simulink model "tesys_original"  (R2020b)
settings: Solver=VariableStepAuto  StartTime=0.0  StopTime=100  RelTol=1e-3
values from neighbouring files (symbols this model uses):
  chisqResidualExp = [0.0306450479532 0.0531264498325 0.923642363871 -0.0297874458631 -0.514662448138 -0.00656924053761 -0.0063391426586 0.00645293061692 -0.0736933231173 -0.060106090774 -0.0130451403889 -0.410405834788 ... (256 elements, 16x16)]    [basevars_performanceTests.mat]
  NoiseVariance = [0.018084969162 0.0123441994291 0.623950185025 -0.0183166694842 -0.436214576367 -0.00523694618209 -0.007053197837 0.0054321930422 -0.0564553252382 -0.0606906681254 -0.0118460528722 -0.365322092979 ... (256 elements, 16x16)]    [basevars_performanceTests.mat]
  threshold = 25.9894230826    [basevars_performanceTests.mat]
  u0 = [63.053 53.98 24.644 61.302 22.21 40.064 38.1 46.534 47.446 41.106 18.114 50]    [basevars_performanceTests.mat]
  y0 = [0.250521392428 3664.03885069 4509.26819729 9.3477426267 2704.99998425 74.9999967369 120.399999605 0.337117068415 80.1094039946 50.0000005823 25.1601724781 49.9999996443 ... (16 elements, 16x1)]    [basevars_performanceTests.mat]
undefined symbols (not defined in the file or in its folder): Discrete, sigbuilder_block, ssid_est, ssid_estred, Time
libraries: TElib x17, simulink x1, truetime x1, ctrlSharedLib x1
settings Model: Creator=mazen  LastModifiedBy=mazen
settings DataIOCC: InitialState=xInitialTecode  SaveOperatingPoint=on  SaveFormat=Structure  SaveOutput=off  SaveState=on  SignalLogging=off  DSMLogging=off

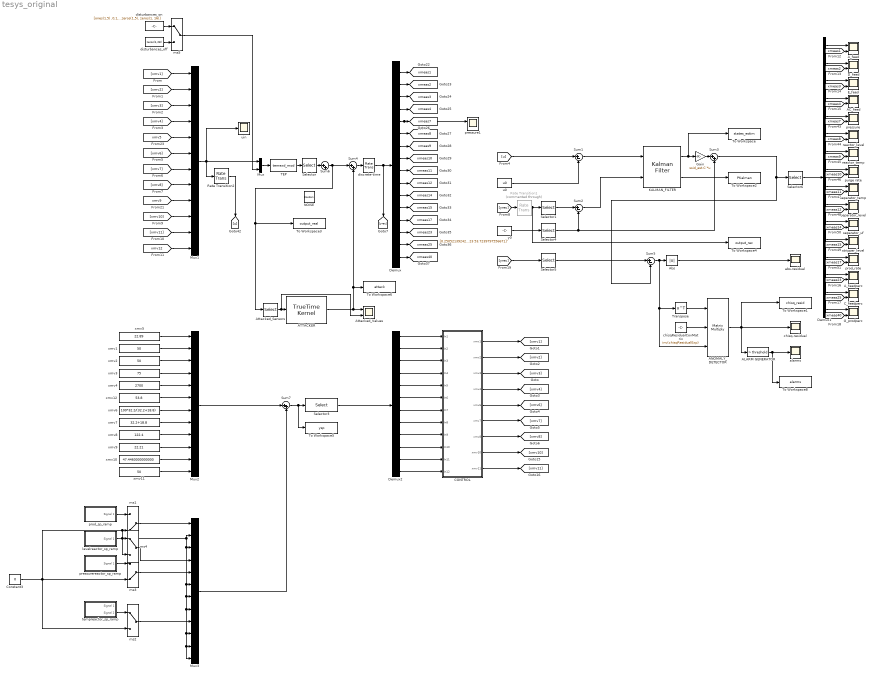
== system tesys_original ==
  AC_feed : Scope  NumInputPorts=2
  ALARM GENERATOR : simulink/Logic and Bit Operations/Compare To Constant  relop=>  const=threshold  OutDataTypeStr=boolean
  ANOMALY_DETECTOR : Product  Inputs=3  Multiplication=Matrix(*)
  ATTACKER : truetime/TrueTime Kernel  sfun=attacker_init  args="struct('FalseAlarmRate',0.1,'Start',20,'AttackedSensors',[5   6   7   9  10  12],'AttackCoef',0.0049316)"  ninputsoutputs=[6 16]  ntriggers=0  trigtype=falling  nwnodenbr=[]  clockoffsetdrift=[0 0]  schedoutput=off  battery=off  poweroutput=off
  A_feed : Scope  NumInputPorts=2
  A_feedperc : Scope  NumInputPorts=2
  Abs : Abs  ZeroCross=off
  Attacked_Sensors : Selector  InputPortWidth=16  IndexOptions=Index vector (dialog)  Indices="[5   6   7   9  10  12]"  OutputSizes=1
  Attacked_Values : Scope  NumInputPorts=2
  CONTROL : Subsystem
  C_feedperc : Scope  NumInputPorts=2
  Constant3 : Constant  Value=0
  D_feed : Scope  NumInputPorts=2
  Demux : Demux  Outputs=16
      settings: DisplayOption=none
  Demux1 : Demux  Outputs=16
      settings: DisplayOption=none
  Demux2 : Demux  Outputs=12
  E_feed : Scope  NumInputPorts=2
  G_prodperc : Scope  NumInputPorts=2
  Gain : Gain  Gain=ssid_est.C  Multiplication=Matrix(K*u)
  KALMAN_FILTER : ctrlSharedLib/Kalman Filter  TimeDomain=Discrete-Time  UseCurrentEstimator=off  ModelSource=LTI State-Space Variable  ModelSourceVariable=ssid_est  A=0.95  B=1  C=1  D=0  NumberOfStates=1  NumberOfInputs=1  NumberOfOutputs=1  InitialEstimateSource=Dialog  X0=0  P0=10  UseK=off  UseGH=off  NumberOfProcessNoiseInputs=1  G=eye(size(ssid_estred.A,1))  TimeInvariantG=on  H=zeros(16,50)  TimeInvariantH=on  Q=diag(ones(size(ssid_est.A,1),1))  TimeInvariantQ=on  R=NoiseVariance  TimeInvariantR=on  N=0  TimeInvariantN=on  AddInputPort=on  AddEnablePort=off  OutputEstimatedY=off  OutputP=on  Ts=-1
      link override MemoryX: InitialCondition="[0.011146   -0.044581   -0.057523    0.064041    0.011425    -0.12859    0.010301   -0.022916    -0.07193   -0.023009   -0.055426    0.037347    0.028076    0.037152    -0.03861     0.02741   -0.018561    0.069301    0.039131   -0.021743   0.0059364    0.075828    0.041172    0.018942   -0.016117     0.12945    -0.05531   -0.047396    0.003457  0.00092852   0.0034323  -0.0053009  6.7113e-05   0.0047184   0.0075023  -0.0024375    0.015481   -0.008098   0.0051102    0.004456    0.010581  -0.0041833     0.02045   -0.015462  -0.0080483   -0.010569  -0.0081562    0.041485    -0.02002    0.026945]"
  Mux : Mux  Inputs=2
  Mux1 : Mux  Inputs=12
  Mux2 : Mux  Inputs=12
  Mux3 : Mux  Inputs=12
  NOISE : RandomNumber  Variance=0.001*y0  SampleTime=5e-4
  Rate Transition1 : RateTransition  Commented=through  InitialCondition=y0  OutPortSampleTime=5e-4
  Rate Transition2 : RateTransition  OutPortSampleTime=5e-4
  Selector : Selector  InputPortWidth=41  IndexOptions=Index vector (dialog)  Indices=[1:4, 7:12, 14, 15, 17, 23, 25, 40]  OutputSizes=1
  Selector1 : Selector  InputPortWidth=16  IndexOptions=Index vector (dialog)  Indices=y0_selected  OutputSizes=1
  Selector3 : Selector  InputPortWidth=12  IndexOptions=Index vector (dialog)  Indices=[1,6,7,8,5,3,2,9,4,10,11,12]  OutputSizes=1
  Selector4 : Selector  InputPortWidth=16  IndexOptions=Index vector (dialog)  Indices=y0_selected  OutputSizes=1
  Selector5 : Selector  InputPortWidth=16  IndexOptions=Index vector (dialog)  Indices=y0_selected  OutputSizes=1
  Selector6 : Selector  InputPortWidth=16  IndexOptions=Index vector (dialog)  Indices=y0_selectedinv  OutputSizes=1
  Sum1 : Sum  Inputs=|+-
  Sum2 : Sum  Inputs=|+-
  Sum{3..4,6..7} (4 alike) : Sum  Inputs=|++
  Sum5 : Sum  Inputs=|+-
  TEP : S-Function  FunctionName=temexd_mod  Parameters=[],[], 0  SFunctionDeploymentMode=off  EnableBusSupport=off
  To Workspace : ToWorkspace  VariableName=states_estim  SampleTime=0.01
  To Workspace1 : ToWorkspace  VariableName=chisq_resid  SampleTime=0.01
  To Workspace2 : ToWorkspace  VariableName=PKalman  SampleTime=0.01
  To Workspace3 : ToWorkspace  VariableName=output_real  SampleTime=0.01
  To Workspace4 : ToWorkspace  VariableName=output_rec  SampleTime=0.01
  To Workspace5 : ToWorkspace  VariableName=ysp  SampleTime=0.01
  To Workspace6 : ToWorkspace  VariableName=attack  SampleTime=5e-4
  To Workspace8 : ToWorkspace  VariableName=alarms  SampleTime=5e-4
  Transpose : Math  Operator=transpose  SaturateOnIntegerOverflow=on
  abs-residual : Scope
  alarms : Scope
  chisq-residual : Scope
  chisqResidualCovMatrix : Constant  Value=inv(chisqResidualExp)
  discrete-time : RateTransition  OutPortSampleTime=5e-4
  disturbances_off : Constant  Value=zeros(1,28)
  disturbances_on : Constant  Value=[ones(1,5) ,0,1,zeros(1,5), zeros(1, 16)]
  levelreactor_sp_ramp : Subsystem  Tag=STV Subsys  LoadFcn=sigbuilder_block('load');  StartFcn=sigbuilder_block('start');  StopFcn=sigbuilder_block('stop');  ClipboardFcn=sigbuilder_block('clipboard');  mask(Sigbuilder block){tuvar=[0:10]}
      mask help: Simulink:masks:SigbuilderBlock_MD
      mask init:
      | if ~strcmp(get_param(bdroot(gcbh),'SimulationStatus'),'stopped') tuvar = sigbuilder_block('maskInit'); end
      settings: CopyFcn=sigbuilder_block('copy');  DeleteFcn=sigbuilder_block('delete');  ModelCloseFcn=sigbuilder_block('modelClose');  PreSaveFcn=sigbuilder_block('preSave');  PauseFcn=sigbuilder_block('pause');  ContinueFcn=sigbuilder_block('continue');  NameChangeFcn=sigbuilder_block('namechange');  OpenFcn=sigbuilder_block('open',[437.6 199.2 550.4 400 ]);  CloseFcn=sigbuilder_block('close');
      mask Display: plot(0, 0, 100, 100,[2, 2, 32, 32, 2], [68, 8, 8, 68, 68],[32, 2], [38, 38], [32, 19, 2],[53, 60, 44], [32, 17, 17, 2],[16, 16, 31, 31]);txt = getActiveGroup(gcbh);text(2, 100, txt,'verticalAlignment', 'top');
  ms1 : ManualSwitch  CurrentSetting=0
  ms2 : ManualSwitch
  ms3 : ManualSwitch  CurrentSetting=0
  ms4 : ManualSwitch
  ms5 : ManualSwitch
  pressure : Scope  NumInputPorts=2
  pressure1 : Scope  NumInputPorts=2
  pressurereactor_sp_ramp : Subsystem  Tag=STV Subsys  LoadFcn=sigbuilder_block('load');  StartFcn=sigbuilder_block('start');  StopFcn=sigbuilder_block('stop');  ClipboardFcn=sigbuilder_block('clipboard');  mask(Sigbuilder block){tuvar=[0:10]}
      mask help: Simulink:masks:SigbuilderBlock_MD
      mask init:
      | if ~strcmp(get_param(bdroot(gcbh),'SimulationStatus'),'stopped') tuvar = sigbuilder_block('maskInit'); end
      settings: CopyFcn=sigbuilder_block('copy');  DeleteFcn=sigbuilder_block('delete');  ModelCloseFcn=sigbuilder_block('modelClose');  PreSaveFcn=sigbuilder_block('preSave');  PauseFcn=sigbuilder_block('pause');  ContinueFcn=sigbuilder_block('continue');  NameChangeFcn=sigbuilder_block('namechange');  OpenFcn=sigbuilder_block('open',[437.6 199.2 550.4 400 ]);  CloseFcn=sigbuilder_block('close');
      mask Display: plot(0, 0, 100, 100,[2, 2, 32, 32, 2], [68, 8, 8, 68, 68],[32, 2], [38, 38], [32, 19, 2],[53, 60, 44], [32, 17, 17, 2],[16, 16, 31, 31]);txt = getActiveGroup(gcbh);text(2, 100, txt,'verticalAlignment', 'top');
  prod_rate : Scope  NumInputPorts=2
  prod_sp_ramp : Subsystem  Tag=STV Subsys  LoadFcn=sigbuilder_block('load');  StartFcn=sigbuilder_block('start');  StopFcn=sigbuilder_block('stop');  ClipboardFcn=sigbuilder_block('clipboard');  mask(Sigbuilder block){tuvar=[0:10]}
      mask help: Simulink:masks:SigbuilderBlock_MD
      mask init:
      | if ~strcmp(get_param(bdroot(gcbh),'SimulationStatus'),'stopped') tuvar = sigbuilder_block('maskInit'); end
      settings: CopyFcn=sigbuilder_block('copy');  DeleteFcn=sigbuilder_block('delete');  ModelCloseFcn=sigbuilder_block('modelClose');  PreSaveFcn=sigbuilder_block('preSave');  PauseFcn=sigbuilder_block('pause');  ContinueFcn=sigbuilder_block('continue');  NameChangeFcn=sigbuilder_block('namechange');  OpenFcn=sigbuilder_block('open',[437.6 199.2 550.4 400 ]);  CloseFcn=sigbuilder_block('close');
      mask Display: plot(0, 0, 100, 100,[2, 2, 32, 32, 2], [68, 8, 8, 68, 68],[32, 2], [38, 38], [32, 19, 2],[53, 60, 44], [32, 17, 17, 2],[16, 16, 31, 31]);txt = getActiveGroup(gcbh);text(2, 100, txt,'verticalAlignment', 'top');
  purge rate : Scope  NumInputPorts=2
  reactor_level : Scope  NumInputPorts=2
  reactor_temp : Scope  NumInputPorts=2
  separator_level : Scope  NumInputPorts=2
  separator_temp : Scope  NumInputPorts=2
  separator_uf : Scope  NumInputPorts=2
  stripper_level : Scope  NumInputPorts=2
  tempreactor_sp_ramp : Subsystem  Tag=STV Subsys  LoadFcn=sigbuilder_block('load');  StartFcn=sigbuilder_block('start');  StopFcn=sigbuilder_block('stop');  ClipboardFcn=sigbuilder_block('clipboard');  mask(Sigbuilder block){tuvar=[0:10]}
      mask help: Simulink:masks:SigbuilderBlock_MD
      mask init:
      | if ~strcmp(get_param(bdroot(gcbh),'SimulationStatus'),'stopped') tuvar = sigbuilder_block('maskInit'); end
      settings: CopyFcn=sigbuilder_block('copy');  DeleteFcn=sigbuilder_block('delete');  ModelCloseFcn=sigbuilder_block('modelClose');  PreSaveFcn=sigbuilder_block('preSave');  PauseFcn=sigbuilder_block('pause');  ContinueFcn=sigbuilder_block('continue');  NameChangeFcn=sigbuilder_block('namechange');  OpenFcn=sigbuilder_block('open',[437.6 199.2 550.4 400 ]);  CloseFcn=sigbuilder_block('close');
      mask Display: plot(0, 0, 100, 100,[2, 2, 32, 32, 2], [68, 8, 8, 68, 68],[32, 2], [38, 38], [32, 19, 2],[53, 60, 44], [32, 17, 17, 2],[16, 16, 31, 31]);txt = getActiveGroup(gcbh);text(2, 100, txt,'verticalAlignment', 'top');
  u0 : Constant  Value=u0  VectorParams1D=off
  "uin " : Scope
  xmv1 : Constant  Value=50
  xmv10 : Constant  Value=47.4460000000000
  xmv11 : Constant  Value=50
  xmv12 : Constant  Value=53.8
  xmv2 : Constant  Value=50
  xmv3 : Constant  Value=75
  xmv4 : Constant  Value=2700
  xmv5 : Constant  Value=22.89
  xmv6 : Constant  Value=100*32.2/(32.2+18.8)
  xmv7 : Constant  Value=32.2+18.8
  xmv8 : Constant  Value=122.4
  xmv9 : Constant  Value=22.21
  y0 : Constant  Value="[0.250521392427743\t3664.03885068600\t4509.26819729219\t9.34774262670434\t2704.99998424633\t74.9999967369169\t120.399999605037\t0.337117068414812\t80.1094039945582\t50.0000005822578\t25.1601724780539\t49.9999996443422\t22.9487308033689\t32.1876133826046\t26.3832900314723\t53.7239797556671]'"
  tag scope: xmeas10=global, xmeas11=global, xmeas12=global, xmeas14=global, xmeas15=global, xmeas17=global, xmeas1=global, xmeas23=global, xmeas25=global, xmeas2=global, xmeas3=global, xmeas40=global, xmeas4=global, xmeas7=global, xmeas8=global, xmeas9=global
  wires:
  [xmeas14] -> separator_uf/2
  [xmv11] -> Mux1/11
  [xmeas15] -> stripper_level/2
  [xmeas8] -> reactor_level/2
  [xmeas10] -> purge rate/2
  [xmeas11] -> separator_temp/2
  Demux/7 -> [xmeas9]
  Demux/5 -> pressure1/1, [xmeas7]
  Demux/9 -> [xmeas11]
  [xmeas12] -> separator_level/2
  [xmeas9] -> reactor_temp/2
  Sum6/1 -> Sum4/1, To Workspace3/1, Attacked_Sensors/1
  [xmv1] -> Mux1/1
  [xmv7] -> Mux1/7
  discrete-time/1 -> Demux/1, [yrec]
  [xmv10] -> Mux1/10
  [xmv8] -> Mux1/8
  [xmv6] -> Mux1/6
  Demux/6 -> [xmeas8]
  TEP/1 -> Selector/1
  [xmv5] -> Mux1/5
  [xmv3] -> Mux1/3
  [xmv4] -> Mux1/4
  Mux/1 -> TEP/1
  [xmeas7] -> pressure/2
  [xmeas17] -> prod_rate/2
  [xmv2] -> Mux1/2
  Demux/16 -> [xmeas40]
  Demux/15 -> [xmeas25]
  Demux/13 -> [xmeas17]
  Demux/11 -> [xmeas14]
  Demux/1 -> [xmeas1]
  Demux/3 -> [xmeas3]
  Demux/10 -> [xmeas12]
  u0/1 -> Sum1/2
  Demux/12 -> [xmeas15]
  [u] -> Sum1/1
  [xmv12] -> Mux1/12
  ms5/1 -> Mux/2
  [xmv9] -> Mux1/9
  Demux/4 -> [xmeas4]
  KALMAN_FILTER/1 -> Gain/1, To Workspace/1
  Demux/8 -> [xmeas10]
  y0/1 -> Selector4/1
  Demux/14 -> [xmeas23]
  Gain/1 -> Sum3/1
  xmv7/1 -> Mux2/8
  xmv12/1 -> Mux2/6
  xmv11/1 -> Mux2/12
  xmv4/1 -> Mux2/5
  Mux3/1 -> Sum7/2
  xmv9/1 -> Mux2/10
  xmv1/1 -> Mux2/2
  Sum7/1 -> To Workspace5/1, Selector3/1
  xmv8/1 -> Mux2/9
  xmv5/1 -> Mux2/1
  Mux2/1 -> Sum7/1
  xmv6/1 -> Mux2/7
  xmv2/1 -> Mux2/3
  xmv3/1 -> Mux2/4
  xmv10/1 -> Mux2/11
  ms1/1 -> Mux3/1
  ms2/1 -> Mux3/9
  levelreactor_sp_ramp/1(Signal 1) -> ms4/1
  ms3/1 -> Mux3/5
  pressurereactor_sp_ramp/1(Signal 1) -> ms3/1
  tempreactor_sp_ramp/2(Signal 2) -> ms2/1
  ms4/1 -> Mux3/4
  Constant3/1 -> ms3/2, ms2/2, Mux3/12, Mux3/11, Mux3/10, Mux3/8, Mux3/7, Mux3/6, Mux3/3, Mux3/2, ms4/2, ms1/2
  prod_sp_ramp/1(Signal 1) -> ms1/1
  Selector3/1 -> Demux2/1
  Demux2/1 -> CONTROL/1(In1)
  Demux2/2 -> CONTROL/2(In2)
  Demux2/3 -> CONTROL/3(In3)
  Demux2/4 -> CONTROL/4(In4)
  Demux2/5 -> CONTROL/5(In5)
  Demux2/6 -> CONTROL/6(In6)
  Demux2/7 -> CONTROL/7(In7)
  Demux2/8 -> CONTROL/8(In8)
  Demux2/9 -> CONTROL/9(In9)
  Demux2/10 -> CONTROL/10(In10)
  Demux2/11 -> CONTROL/11(In11)
  Demux2/12 -> CONTROL/12(In12)
  CONTROL/1(xmv1) -> [xmv1]
  CONTROL/2(xmv2) -> [xmv2]
  CONTROL/3(xmv3) -> [xmv3]
  CONTROL/4(xmv4) -> [xmv4]
  CONTROL/5(xmv6) -> [xmv6]
  CONTROL/6(xmv7) -> [xmv7]
  CONTROL/7(xmv8) -> [xmv8]
  CONTROL/8(xmv10) -> [xmv10]
  CONTROL/9(xmv11) -> [xmv11]
  Demux1/5 -> pressure/1
  Demux1/6 -> reactor_level/1
  Demux1/7 -> reactor_temp/1
  Demux1/9 -> separator_temp/1
  Demux1/10 -> separator_level/1
  Demux1/11 -> separator_uf/1
  Demux1/12 -> stripper_level/1
  Demux1/13 -> prod_rate/1
  Demux1/8 -> purge rate/1
  Sum5/1 -> ANOMALY_DETECTOR/3, Transpose/1, Abs/1
  ANOMALY_DETECTOR/1 -> ALARM GENERATOR/1, chisq-residual/1, To Workspace1/1
  Transpose/1 -> ANOMALY_DETECTOR/1
  Abs/1 -> abs-residual/1
  Rate Transition1/1 -> To Workspace4/1, Selector1/1
  Demux/2 -> [xmeas2]
  Demux1/1 -> A_feed/1
  [xmeas1] -> A_feed/2
  Demux1/2 -> D_feed/1
  [xmeas2] -> D_feed/2
  Demux1/3 -> E_feed/1
  [xmeas3] -> E_feed/2
  Demux1/4 -> AC_feed/1
  [xmeas4] -> AC_feed/2
  Demux1/14 -> A_feedperc/1
  [xmeas23] -> A_feedperc/2
  Demux1/15 -> C_feedperc/1
  [xmeas25] -> C_feedperc/2
  Demux1/16 -> G_prodperc/1
  [xmeas40] -> G_prodperc/2
  chisqResidualCovMatrix/1 -> ANOMALY_DETECTOR/2
  ALARM GENERATOR/1 -> To Workspace8/1, alarms/1
  Sum2/1 -> KALMAN_FILTER/2
  Sum3/1 -> Selector6/1, Sum5/2
  Mux1/1 -> Mux/1, "uin "/1, Rate Transition2/1
  Sum1/1 -> KALMAN_FILTER/1
  Selector/1 -> Sum6/1
  [yrec] -> Selector5/1
  Sum4/1 -> discrete-time/1
  [yrec] -> Rate Transition1/1
  Attacked_Sensors/1 -> Attacked_Values/2, ATTACKER/1
  ATTACKER/1 -> Sum4/2, To Workspace6/1, Attacked_Values/1
  disturbances_on/1 -> ms5/1
  disturbances_off/1 -> ms5/2
  Selector1/1 -> Sum2/1
  Selector4/1 -> Sum2/2, Sum3/2
  Selector5/1 -> Sum5/1
  Selector6/1 -> Demux1/1
  Rate Transition2/1 -> [u]
  KALMAN_FILTER/2 -> To Workspace2/1

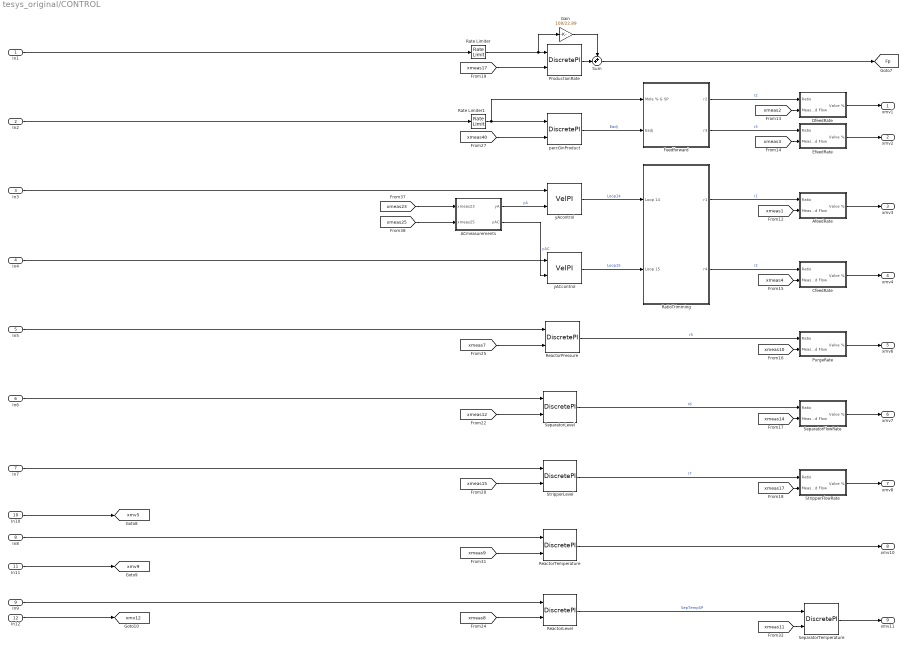
== system tesys_original/CONTROL ==
  In1 : Inport
  In2 : Inport  Port=2
  In3 : Inport  Port=3
  In4 : Inport  Port=4
  In5 : Inport  Port=5
  In6 : Inport  Port=6
  In7 : Inport  Port=7
  In8 : Inport  Port=8
  In9 : Inport  Port=9
  In10 : Inport  Port=10
  In11 : Inport  Port=11
  In12 : Inport  Port=12
  ACmeasurements : Subsystem
  AfeedRate : Subsystem
  CfeedRate : Subsystem
  DfeedRate : Subsystem
  EfeedRate : Subsystem
  Feedforward : Subsystem
  Gain : Gain  Gain=100/22.89  SaturateOnIntegerOverflow=on  OutDataTypeStr=Inherit: Same as input  ParamDataTypeStr=Inherit: Same as input
  ProductionRate : TElib/DiscretePI  Kc=3.2  Ti=120/60  Ts=5e-4  x0=100  Hi=30  Lo=-30
  PurgeRate : Subsystem
  Rate Limiter : RateLimiter  RisingSlewLimit=0.3*22.95/24  FallingSlewLimit=-0.3*22.95/24
  Rate Limiter1 : RateLimiter  RisingSlewLimit=50/24  FallingSlewLimit=-50/24
  RatioTrimming : Subsystem
  ReactorLevel : TElib/DiscretePI  Kc=0.8  Ti=60/60  Ts=5e-4  x0=80.100000000000000  Hi=120  Lo=0
  ReactorPressure : TElib/DiscretePI  Kc=-1e-4  Ti=20/60  Ts=5e-4  x0=0.003370000000000  Hi=100  Lo=0
  ReactorTemperature : TElib/DiscretePI  Kc=-8  Ti=7.5/60  Ts=5e-4  x0=41.106000000000000  Hi=100  Lo=0
  SeparatorFlowRate : Subsystem
  SeparatorLevel : TElib/DiscretePI  Kc=-1e-3  Ti=200/60  Ts=5e-4  x0=0.251600000000000  Hi=100  Lo=0
  SeparatorTemperature : TElib/DiscretePI  Kc=-4  Ti=15/60  Ts=5e-4  x0=18.114000000000000  Hi=100  Lo=0
  StripperFlowRate : Subsystem
  StripperLevel : TElib/DiscretePI  Kc=-2e-4  Ti=200/60  Ts=5e-4  x0=0.229500000000000  Hi=100  Lo=0
  Sum : Sum  Inputs=++|  SaturateOnIntegerOverflow=on
  percGinProduct : TElib/DiscretePI  Kc=-0.4  Ti=100/60  Ts=5e-4  x0=0  Hi=inf  Lo=-inf
  yACcontrol : TElib/DiscretePI/VelPI  Kc=3e-4  Ti=2  Ts=0.1
  yAcontrol : TElib/DiscretePI/VelPI  Kc=2e-4  Ti=1  Ts=0.1
  xmv1 : Outport
  xmv2 : Outport  Port=2
  xmv3 : Outport  Port=3
  xmv4 : Outport  Port=4
  xmv6 : Outport  Port=5
  xmv7 : Outport  Port=6
  xmv8 : Outport  Port=7
  xmv10 : Outport  Port=8
  xmv11 : Outport  Port=9
  tag scope: Fp=global, xmv12=global, xmv5=global, xmv9=global
  wires:
  In6/1 -> SeparatorLevel/1
  yAcontrol/1 -> RatioTrimming/1(Loop 14)  "Loop14"
  Rate Limiter/1 -> ProductionRate/1, Gain/1
  [xmeas1] -> AfeedRate/2(Measured Flow)
  [xmeas10] -> PurgeRate/2(Measured Flow)
  ReactorLevel/1 -> SeparatorTemperature/1  "SepTempSP"
  [xmeas17] -> ProductionRate/2
  In10/1 -> [xmv5]
  AfeedRate/1(Valve %) -> xmv3/1
  RatioTrimming/2(r4) -> CfeedRate/1(Ratio)  "r2"
  percGinProduct/1 -> Feedforward/2(Eadj)  "Eadj"
  Feedforward/1(r2) -> DfeedRate/1(Ratio)  "r2"
  ReactorTemperature/1 -> xmv10/1
  In1/1 -> Rate Limiter/1
  RatioTrimming/1(r1) -> AfeedRate/1(Ratio)  "r1"
  EfeedRate/1(Valve %) -> xmv2/1
  SeparatorTemperature/1 -> xmv11/1
  In2/1 -> Rate Limiter1/1
  [xmeas40] -> percGinProduct/2
  [xmeas25] -> ACmeasurements/2(xmeas25)
  In7/1 -> StripperLevel/1
  ACmeasurements/2(yAC) -> yACcontrol/2  "yAC"
  yACcontrol/1 -> RatioTrimming/2(Loop 15)  "Loop15"
  ACmeasurements/1(yA) -> yAcontrol/2  "yA"
  SeparatorFlowRate/1(Valve %) -> xmv7/1
  ProductionRate/1 -> Sum/2
  Gain/1 -> Sum/1
  [xmeas3] -> EfeedRate/2(Measured Flow)
  [xmeas23] -> ACmeasurements/1(xmeas23)
  [xmeas15] -> StripperLevel/2
  [xmeas9] -> ReactorTemperature/2
  In12/1 -> [xmv12]
  StripperLevel/1 -> StripperFlowRate/1(Ratio)  "r7"
  SeparatorLevel/1 -> SeparatorFlowRate/1(Ratio)  "r6"
  Rate Limiter1/1 -> Feedforward/1(Mole % G SP), percGinProduct/1
  Sum/1 -> [Fp]
  Feedforward/2(r3) -> EfeedRate/1(Ratio)  "r3"
  DfeedRate/1(Valve %) -> xmv1/1
  [xmeas12] -> SeparatorLevel/2
  [xmeas2] -> DfeedRate/2(Measured Flow)
  [xmeas17] -> StripperFlowRate/2(Measured Flow)
  [xmeas4] -> CfeedRate/2(Measured Flow)
  In9/1 -> ReactorLevel/1
  [xmeas8] -> ReactorLevel/2
  ReactorPressure/1 -> PurgeRate/1(Ratio)  "r5"
  [xmeas14] -> SeparatorFlowRate/2(Measured Flow)
  [xmeas7] -> ReactorPressure/2
  PurgeRate/1(Valve %) -> xmv6/1
  [xmeas11] -> SeparatorTemperature/2
  In8/1 -> ReactorTemperature/1
  StripperFlowRate/1(Valve %) -> xmv8/1
  CfeedRate/1(Valve %) -> xmv4/1
  In3/1 -> yAcontrol/1
  In5/1 -> ReactorPressure/1
  In4/1 -> yACcontrol/1
  In11/1 -> [xmv9]

== system tesys_original/levelreactor_sp_ramp ==
  Demux : Demux  Tag=STV Demux  Outputs=1
      settings: DisplayOption=none
  FromWs : FromWorkspace  Tag=STV FromWs  VariableName=tuvar
      SigBuilderData=|
      | common.afterFinalStr = 'Extrapolate'
      | common.sampleTime = 0
      | dataSet.timeRange = [0 300]
      | dataSet.name = 'Group 1'
      | sbobj.Groups.Name = 'Group 1'
      | sbobj.Groups.Signals.Name = 'Signal 1'
      | sbobj.Groups.Signals.XData = [0 10 100 200 300]
      | sbobj.Groups.Signals.YData = [0 -2.2 -20 -14.8 -14.8]
      | sbobj.Groups.TimeRange = [0 300]
  Signal 1 : Outport  Tag=STV Outport
  wires:
  Demux/1 -> Signal 1/1
  FromWs/1 -> Demux/1

== system tesys_original/pressurereactor_sp_ramp ==
  Demux : Demux  Tag=STV Demux  Outputs=1
      settings: DisplayOption=none
  FromWs : FromWorkspace  Tag=STV FromWs  VariableName=tuvar
      SigBuilderData=|
      | common.afterFinalStr = 'Extrapolate'
      | common.sampleTime = 0
      | dataSet.timeRange = [0 500]
      | dataSet.name = 'Group 1'
      | sbobj.Groups.Name = 'Group 1'
      | sbobj.Groups.Signals.Name = 'Signal 1'
      | sbobj.Groups.Signals.XData = [0 10 100 270 270 300 300 500]
      | sbobj.Groups.Signals.YData = [0 0 200 16 260 260 256 256]
      | sbobj.Groups.TimeRange = [0 500]
  Signal 1 : Outport  Tag=STV Outport
  wires:
  Demux/1 -> Signal 1/1
  FromWs/1 -> Demux/1

== system tesys_original/prod_sp_ramp ==
  Demux : Demux  Tag=STV Demux  Outputs=1
      settings: DisplayOption=none
  FromWs : FromWorkspace  Tag=STV FromWs  VariableName=tuvar
      SigBuilderData=|
      | common.afterFinalStr = 'Extrapolate'
      | common.sampleTime = 0
      | dataSet.timeRange = [0 300]
      | dataSet.name = 'Group 1'
      | sbobj.Groups.Name = 'Group 1'
      | sbobj.Groups.Signals.Name = 'Signal 1'
      | sbobj.Groups.Signals.XData = [0 100 200 200 300]
      | sbobj.Groups.Signals.YData = [0 8 8.1 8.05 8.05]
      | sbobj.Groups.TimeRange = [0 300]
  Signal 1 : Outport  Tag=STV Outport
  wires:
  Demux/1 -> Signal 1/1
  FromWs/1 -> Demux/1

== system tesys_original/tempreactor_sp_ramp ==
  Demux : Demux  Tag=STV Demux  Outputs=2
      settings: DisplayOption=none
  FromWs : FromWorkspace  Tag=STV FromWs  VariableName=tuvar
      SigBuilderData=|
      | common.afterFinalStr = 'Extrapolate'
      | common.sampleTime = 0
      | dataSet.timeRange = [0 300]
      | dataSet.name = 'Group 1'
      | sbobj.Groups.Name = 'Group 1'
      | sbobj.Groups.Signals(1).Name = 'Signal 1'
      | sbobj.Groups.Signals(1).XData = [0 20 200 200 300]
      | sbobj.Groups.Signals(1).YData = [0 -15 -15.2 -20 15]
      | sbobj.Groups.Signals(2).Name = 'Signal 2'
      | sbobj.Groups.Signals(2).XData = [0 300]
      | sbobj.Groups.Signals(2).YData = [0 0]
      | sbobj.Groups.TimeRange = [0 300]
  Signal 1 : Outport  Tag=STV Outport
  Signal 2 : Outport  Tag=STV Outport  Port=2
  wires:
  Demux/1 -> Signal 1/1
  FromWs/1 -> Demux/1
  Demux/2 -> Signal 2/1

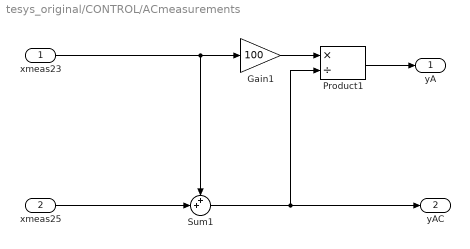
== system tesys_original/CONTROL/ACmeasurements ==
  xmeas23 : Inport
  xmeas25 : Inport  Port=2
  Gain1 : Gain  Gain=100  SaturateOnIntegerOverflow=on  OutDataTypeStr=Inherit: Same as input  ParamDataTypeStr=Inherit: Same as input
  Product1 : Product  Inputs=*/  SaturateOnIntegerOverflow=on  OutDataTypeStr=Inherit: Same as first input
  Sum1 : Sum  Inputs=++|  SaturateOnIntegerOverflow=on
  yA : Outport
  yAC : Outport  Port=2
  wires:
  Sum1/1 -> yAC/1, Product1/2
  xmeas23/1 -> Sum1/1, Gain1/1
  xmeas25/1 -> Sum1/2
  Gain1/1 -> Product1/1
  Product1/1 -> yA/1

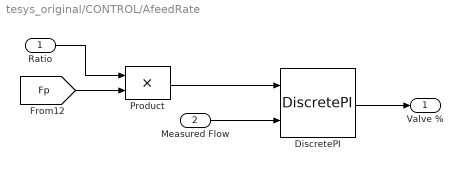
== system tesys_original/CONTROL/AfeedRate ==
  Ratio : Inport
  Measured Flow : Inport  Port=2
  DiscretePI : TElib/DiscretePI  Kc=0.01  Ti=0.001/60  Ts=5e-4  x0=24.644000000000000  Hi=100  Lo=0
  Product : Product  SaturateOnIntegerOverflow=on  OutDataTypeStr=Inherit: Same as first input
  Valve % : Outport
  wires:
  DiscretePI/1 -> Valve %/1
  Ratio/1 -> Product/1
  [Fp] -> Product/2
  Measured Flow/1 -> DiscretePI/2
  Product/1 -> DiscretePI/1

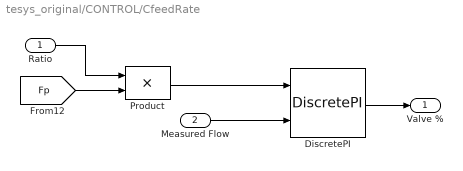
== system tesys_original/CONTROL/CfeedRate ==
  Ratio : Inport
  Measured Flow : Inport  Port=2
  DiscretePI : TElib/DiscretePI  Kc=0.003  Ti=0.001/60  Ts=5e-4  x0=61.302000000000000  Hi=100  Lo=0
  Product : Product  SaturateOnIntegerOverflow=on  OutDataTypeStr=Inherit: Same as first input
  Valve % : Outport
  wires:
  Product/1 -> DiscretePI/1
  Measured Flow/1 -> DiscretePI/2
  [Fp] -> Product/2
  Ratio/1 -> Product/1
  DiscretePI/1 -> Valve %/1

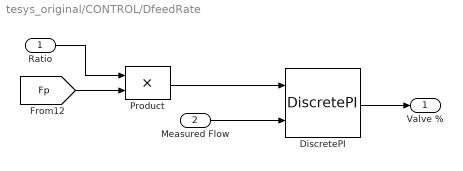
== system tesys_original/CONTROL/DfeedRate ==
  Ratio : Inport
  Measured Flow : Inport  Port=2
  DiscretePI : TElib/DiscretePI  Kc=1.6e-6  Ti=0.001/60  Ts=5e-4  x0=63.053000000000000  Hi=100  Lo=0
  Product : Product  SaturateOnIntegerOverflow=on  OutDataTypeStr=Inherit: Same as first input
  Valve % : Outport
  wires:
  Product/1 -> DiscretePI/1
  Measured Flow/1 -> DiscretePI/2
  [Fp] -> Product/2
  Ratio/1 -> Product/1
  DiscretePI/1 -> Valve %/1

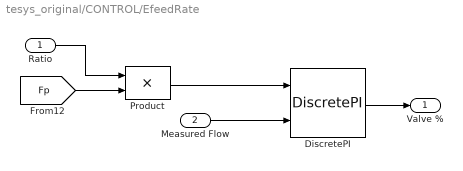
== system tesys_original/CONTROL/EfeedRate ==
  Ratio : Inport
  Measured Flow : Inport  Port=2
  DiscretePI : TElib/DiscretePI  Kc=1.8e-6  Ti=0.001/60  Ts=5e-4  x0=53.980000000000000  Hi=100  Lo=0
  Product : Product  SaturateOnIntegerOverflow=on  OutDataTypeStr=Inherit: Same as first input
  Valve % : Outport
  wires:
  Product/1 -> DiscretePI/1
  Measured Flow/1 -> DiscretePI/2
  [Fp] -> Product/2
  Ratio/1 -> Product/1
  DiscretePI/1 -> Valve %/1

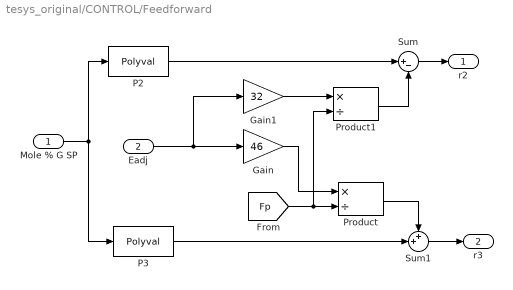
== system tesys_original/CONTROL/Feedforward ==
  Mole % G SP : Inport
  Eadj : Inport  Port=2
  Gain : Gain  Gain=46  SaturateOnIntegerOverflow=on  OutDataTypeStr=Inherit: Same as input  ParamDataTypeStr=Inherit: Same as input
  Gain1 : Gain  Gain=32  SaturateOnIntegerOverflow=on  OutDataTypeStr=Inherit: Same as input  ParamDataTypeStr=Inherit: Same as input
  P2 : Polyval  Coefs="[1.5192e-003  5.9446e-001  2.7690e-001]"
  P3 : Polyval  Coefs="[-1.1377e-003 -8.0893e-001  9.1060e+001]"
  Product : Product  Inputs=*/  SaturateOnIntegerOverflow=on  OutDataTypeStr=Inherit: Same as first input
  Product1 : Product  Inputs=*/  SaturateOnIntegerOverflow=on  OutDataTypeStr=Inherit: Same as first input
  Sum : Sum  Inputs=|+-  SaturateOnIntegerOverflow=on
  Sum1 : Sum  Inputs=++|  SaturateOnIntegerOverflow=on
  r2 : Outport
  r3 : Outport  Port=2
  wires:
  Mole % G SP/1 -> P2/1, P3/1
  Sum/1 -> r2/1
  P2/1 -> Sum/1
  Sum1/1 -> r3/1
  P3/1 -> Sum1/2
  Product/1 -> Sum1/1
  [Fp] -> Product/2, Product1/2
  Gain/1 -> Product/1
  Eadj/1 -> Gain/1, Gain1/1
  Product1/1 -> Sum/2
  Gain1/1 -> Product1/1

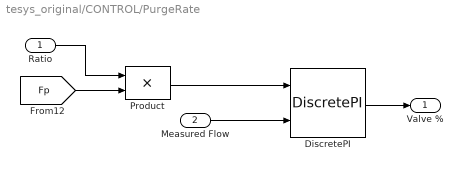
== system tesys_original/CONTROL/PurgeRate ==
  Ratio : Inport
  Measured Flow : Inport  Port=2
  DiscretePI : TElib/DiscretePI  Kc=0.01  Ti=0.001/60  Ts=5e-4  x0=40.064000000000000  Hi=100  Lo=0
  Product : Product  SaturateOnIntegerOverflow=on  OutDataTypeStr=Inherit: Same as first input
  Valve % : Outport
  wires:
  DiscretePI/1 -> Valve %/1
  Ratio/1 -> Product/1
  [Fp] -> Product/2
  Measured Flow/1 -> DiscretePI/2
  Product/1 -> DiscretePI/1

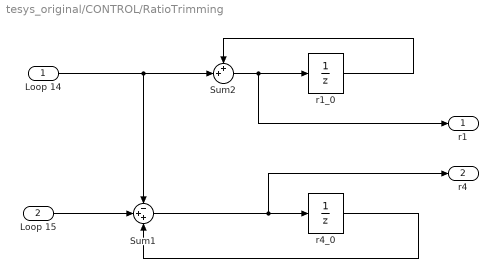
== system tesys_original/CONTROL/RatioTrimming ==
  Loop 14 : Inport
  Loop 15 : Inport  Port=2
  Sum1 : Sum  Inputs=-++  SaturateOnIntegerOverflow=on
  Sum2 : Sum  Inputs=++|  SaturateOnIntegerOverflow=on
  r1_0 : UnitDelay  InitialCondition=0.0043115  SampleTime=0.1  HasFrameUpgradeWarning=on
  r4_0 : UnitDelay  InitialCondition=0.08929  SampleTime=0.1  HasFrameUpgradeWarning=on
  r1 : Outport
  r4 : Outport  Port=2
  wires:
  Loop 15/1 -> Sum1/2
  r1_0/1 -> Sum2/1
  r4_0/1 -> Sum1/3
  Sum2/1 -> r1_0/1, r1/1
  Loop 14/1 -> Sum2/2, Sum1/1
  Sum1/1 -> r4_0/1, r4/1

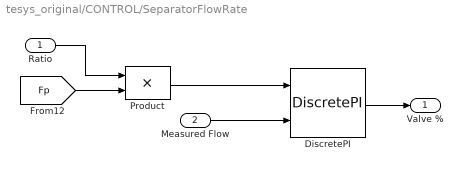
== system tesys_original/CONTROL/SeparatorFlowRate ==
  Ratio : Inport
  Measured Flow : Inport  Port=2
  DiscretePI : TElib/DiscretePI  Kc=4e-4  Ti=0.001/60  Ts=5e-4  x0=38.100000000000000  Hi=100  Lo=0
  Product : Product  SaturateOnIntegerOverflow=on  OutDataTypeStr=Inherit: Same as first input
  Valve % : Outport
  wires:
  Product/1 -> DiscretePI/1
  Measured Flow/1 -> DiscretePI/2
  [Fp] -> Product/2
  Ratio/1 -> Product/1
  DiscretePI/1 -> Valve %/1

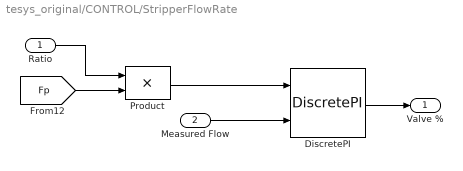
== system tesys_original/CONTROL/StripperFlowRate ==
  Ratio : Inport
  Measured Flow : Inport  Port=2
  DiscretePI : TElib/DiscretePI  Kc=4e-4  Ti=0.001/60  Ts=5e-4  x0=46.534000000000000  Hi=100  Lo=0
  Product : Product  SaturateOnIntegerOverflow=on  OutDataTypeStr=Inherit: Same as first input
  Valve % : Outport
  wires:
  DiscretePI/1 -> Valve %/1
  Ratio/1 -> Product/1
  [Fp] -> Product/2
  Measured Flow/1 -> DiscretePI/2
  Product/1 -> DiscretePI/1
